simulink model "zacc"  (R2020a)
settings: Solver=VariableStepAuto  StartTime=0.0  StopTime=10.0  RelTol=1e-3
undefined symbols (not defined in the file): Az, g, m
settings Model: Creator=Muni Kumar  LastModifiedBy=Muni Kumar

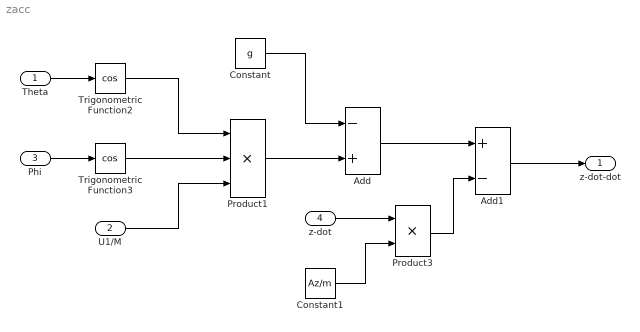
== system zacc ==
  Theta : Inport
  U1/M : Inport  Port=2
  Phi : Inport  Port=3
  z-dot : Inport  Port=4
  Add : Sum  Inputs=-+
  Add1 : Sum  Inputs=+-
  Constant : Constant  Value=g
  Constant1 : Constant  Value=Az/m
  Product1 : Product  Inputs=3
  Product3 : Product
  Trigonometric Function2 : Trigonometry  Operator=cos
  Trigonometric Function3 : Trigonometry  Operator=cos
  z-dot-dot : Outport
  wires:
  Product1/1 -> Add/2
  Theta/1 -> Trigonometric Function2/1
  Trigonometric Function3/1 -> Product1/2
  Add/1 -> Add1/1
  Add1/1 -> z-dot-dot/1
  U1/M/1 -> Product1/3
  Trigonometric Function2/1 -> Product1/1
  Phi/1 -> Trigonometric Function3/1
  Constant/1 -> Add/1
  z-dot/1 -> Product3/1
  Constant1/1 -> Product3/2
  Product3/1 -> Add1/2
